simulink model "simpleFirstOrder"  (R2013a)
settings: Solver=ode4  StartTime=0.0  StopTime=10.0  FixedStep=Ts  RelTol=1e-3
settings Model: Creator=zcarwile  LastModifiedBy=bbhattac
settings OptimizationCC: InlineParams=on  OptimizeModelRefInitCode=on  LifeSpan=1
settings DebuggingCC: ParameterPrecisionLossMsg=none  FcnCallInpInsideContextMsg=UseLocalSettings  StrictBusMsg=Warning
settings RTWCC: SystemTargetFile=ert.tlc  GenCodeOnly=on  TemplateMakefile=ert_default_tmf  Description=Real-Time Workshop Embedded Coder (no auto configuration)  GenerateReport=on  ProcessScript=ert_make_rtw_hook  LaunchReport=on
settings CodeAppCC: IgnoreCustomStorageClasses=off  CustomSymbolStrType=$N$R$M  InternalIdentifier=Classic
settings ERTTargetCC: CombineOutputUpdateFcns=off  SupportContinuousTime=on  InlinedParameterPlacement=Hierarchical  ERTCustomFileTemplate=example_file_process.tlc

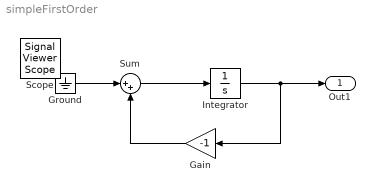
== system simpleFirstOrder ==
  Gain : Gain  Gain=-1
  Ground : Ground
  Integrator : Integrator  InitialCondition=1
  Sum : Sum  Inputs=|++
  Out1 : Outport
  Scope : SignalViewerScope  IOType=viewer  RefreshTime=0.035000
  wires:
  Ground/1 -> Sum/1
  Sum/1 -> Integrator/1
  Gain/1 -> Sum/2
  Integrator/1 -> Out1/1, Gain/1
